simulink model "BCI_Control_Log_2024a"  (R2024a)
settings: Solver=FixedStepAuto  StartTime=0.0  StopTime=inf  FixedStep=1/fs  RelTol=1e-3
InitFcn:
  | RunTime
StopFcn:
  | SaveData
values from neighbouring files (symbols this model uses):
  const_a = Mdl_a.Coeffs(1,2).Const    [RunTime.m]
  ERaw = data{1,1}.X'    [RunTime.m]
  fs = 250    [SaveData.m]    (also in setup.m)
  ind_sel_a = Ia    [OfflineDataAnalysis_Unicorn.m]    (also in RunTime.m = Ia(1:best_feat_a))
  linear_coeffs_a = Mdl_a.Coeffs(1,2).Linear    [RunTime.m]
  shiftLen = 0.20*fs    [RunTime.m]
  winLen = 2*fs    [RunTime.m]
undefined symbols (not defined in the file or in its folder): UN, W1a, W2a
libraries: dspfdesign x34, dspnetwork x4, dspstat3 x2, UnicornLib x1
settings Model: Creator=Utente  LastModifiedBy=IRISc
settings DebuggingCC: UnconnectedInputMsg=warning  UnconnectedOutputMsg=warning  UnconnectedLineMsg=warning
settings ModelReferenceCC: EnableRefExpFcnMdlSchedulingChecks=on
settings RTWCC: GPUComputeCapability=3.5  DLArmComputeVersion=19.05

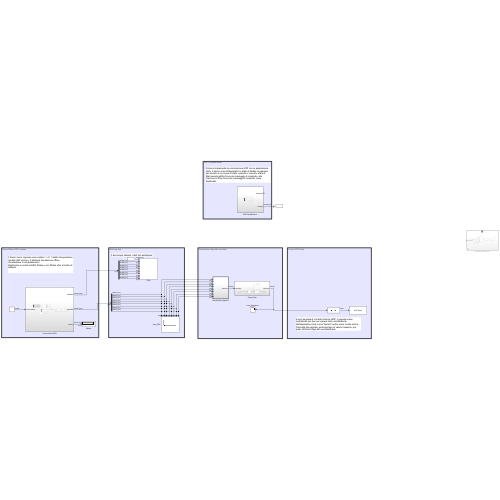
[thumbnail: Simulink's stored preview of the top-level diagram]
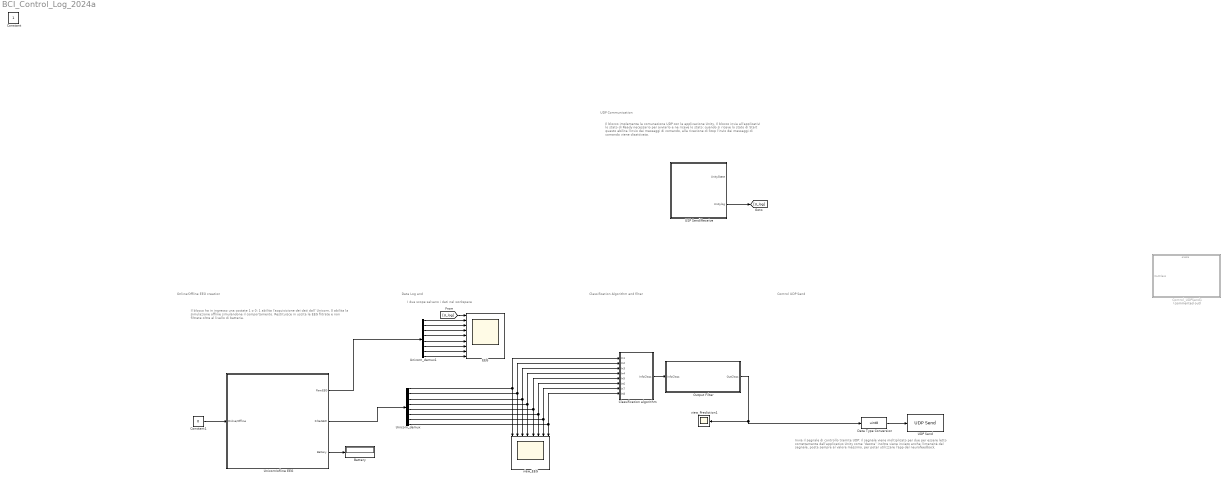
== system BCI_Control_Log_2024a ==
  note: Invia il segnale di controllo tramite UDP: il segnale viene moltiplicato per due per essere letto correttamente dall'applicativo Unity come "destra" inoltre viene inviato anche l'intensità del segnale, posta sempre al valore massimo, per poter utilizzare l'app del neurofeedback.
  note: Control UDP Send
  note: Il blocco implementa la comunazione UDP con le applicazione Unity. Il blocco invia all'applicativi lo stato di Ready necessario per avviarlo e ne riceve lo stato: quando si riceve lo stato di Start questo abilita l'invio dei messaggi di comando, alla ricezione di Stop l'invio dei messaggi di comando viene disattivata.
  note: UDP Communication
  note: Classification Algorithm and filter
  note: I due scope salvano i dati nel workspace
  note: Data Log and
  note: Il blocco ha in ingresso una costate 1 o 0: 1 abilita l'acquisizione dei dati dall' Unicorn, 0 abilita la simulazione offline simulandone il comportamento.
      | Restituisce in uscita le EEG flitrate e non filtrate oltre al livello di batteria.
  note: Online/Offline EEG creation
  Battery : Display
  Classification algorithm : Subsystem  TreatAsAtomicUnit=on
  Constant1 : Constant  Value=0
  Control_UDPSend1 : Subsystem  Commented=on
  Data Type Conversion : DataTypeConversion  OutDataTypeStr=uint8  SaturateOnIntegerOverflow=off  RndMeth=Floor
  EEG : Scope  NumInputPorts=9
  Output Filter : Subsystem
  UDP Send : dspnetwork/UDP Send  remoteURL='127.0.0.1'  remotePort=5010  localURL='0.0.0.0'  localPortSource=Automatically determine  localPort=-1  sendBufferSize=8192  sampletime=-1  blockPlatform=[]  separateLengthPort=0
  "USP Send/Receive " : Subsystem
  Unicorn/ofline EEG : Subsystem
  Unicorn_demux : Demux  Outputs=8
  Unicorn_demux1 : Demux  Outputs=8
  view_EEG : Scope  NumInputPorts=8
  view_Prediction1 : Scope
  Constant : Constant  IOType=siggen
  wires:
  Unicorn_demux/8 -> Classification algorithm/8(In8), view_EEG/8
  Unicorn_demux/7 -> Classification algorithm/7(In7), view_EEG/7
  Unicorn_demux/6 -> Classification algorithm/6(In6), view_EEG/6
  Unicorn_demux/5 -> Classification algorithm/5(In5), view_EEG/5
  Unicorn_demux/4 -> Classification algorithm/4(In4), view_EEG/4
  Unicorn_demux/1 -> Classification algorithm/1(In1), view_EEG/1
  Unicorn_demux/2 -> Classification algorithm/2(In2), view_EEG/2
  Unicorn_demux/3 -> Classification algorithm/3(In3), view_EEG/3
  Classification algorithm/1(InfoClass) -> Output Filter/1(InfoClass)
  Output Filter/1(OutClass) -> Data Type Conversion/1, view_Prediction1/1
  Unicorn/ofline EEG/2(FilterEEG) -> Unicorn_demux/1
  Unicorn/ofline EEG/1(RawEEG) -> Unicorn_demux1/1
  Unicorn/ofline EEG/3(Battery) -> Battery/1
  Constant1/1 -> Unicorn/ofline EEG/1(Online/Offline)
  Unicorn_demux1/1 -> EEG/2
  Unicorn_demux1/2 -> EEG/3
  Unicorn_demux1/3 -> EEG/4
  Unicorn_demux1/4 -> EEG/5
  Unicorn_demux1/5 -> EEG/6
  Unicorn_demux1/6 -> EEG/7
  Unicorn_demux1/7 -> EEG/8
  Unicorn_demux1/8 -> EEG/9
  "USP Send/Receive "/2(Unitylog) -> [U_log]
  [U_log] -> EEG/1
  Data Type Conversion/1 -> UDP Send/1

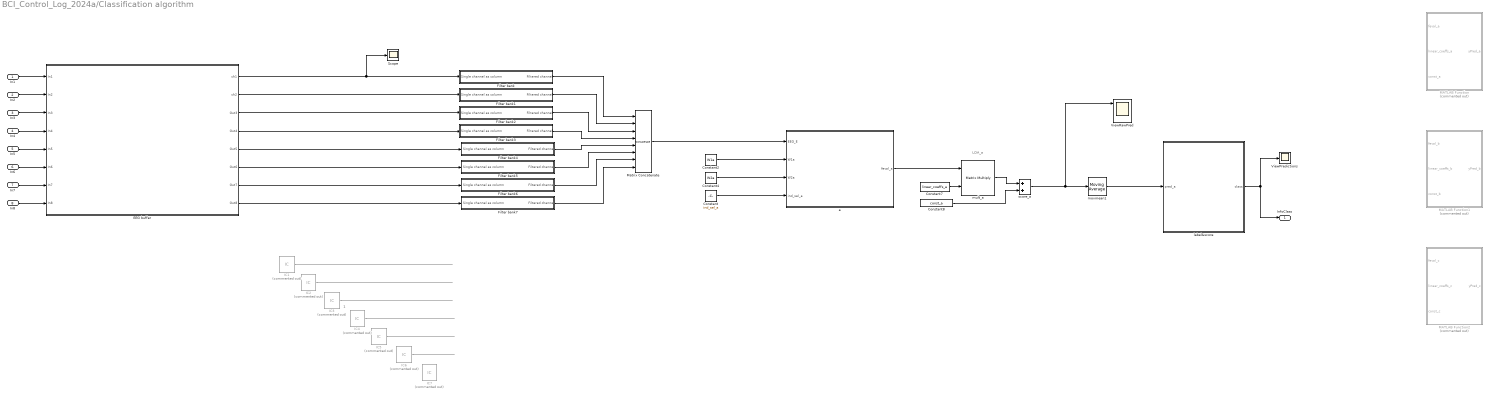
== system BCI_Control_Log_2024a/Classification algorithm ==
  note: LDA_a
  note: 1
  In1 : Inport
  In2 : Inport  Port=2
  In3 : Inport  Port=3
  In4 : Inport  Port=4
  In5 : Inport  Port=5
  In6 : Inport  Port=6
  In7 : Inport  Port=7
  In8 : Inport  Port=8
  Constant : Constant  Value=ind_sel_a
  Constant2 : Constant  Value=W1a
  Constant4 : Constant  Value=W2a
  Constant7 : Constant  Value=linear_coeffs_a
  Constant8 : Constant  Value=const_a
  EEG buffer : Subsystem
  Filter bank : Subsystem
  Filter bank1 : Subsystem
  Filter bank2 : Subsystem
  Filter bank3 : Subsystem
  Filter bank4 : Subsystem
  Filter bank5 : Subsystem
  Filter bank6 : Subsystem
  Filter bank7 : Subsystem
  IC{1..7} (7 alike) : InitialCondition  Commented=on  Value=0.1
  MATLAB Function : MATLAB Function  Commented=on  TreatAsAtomicUnit=on
  MATLAB Function1 : MATLAB Function  Commented=on  TreatAsAtomicUnit=on
  MATLAB Function2 : MATLAB Function  Commented=on  TreatAsAtomicUnit=on
  Matrix Concatenate : Concatenate  NumInputs=8  Mode=Multidimensional array  ConcatenateDimension=3
  Scope : Scope
  ViewPredictions : Scope
  ViewRawPred : Scope  NumInputPorts=3
  a : MATLAB Function  TreatAsAtomicUnit=on
  label&score : MATLAB Function  TreatAsAtomicUnit=on
  movmean1 : dspstat3/Moving Average  Method=Sliding window  ForgettingFactorPort=off  SpecifyWindowLength=on  WindowLength=3  OverlapLength=2  AllowArbitraryInputLength=off  ForgettingFactor=0.9  SimulateUsing=Code generation
  mult_a : Product  Multiplication=Matrix(*)
  score_a : Sum
  InfoClass : Outport
  wires:
  In1/1 -> EEG buffer/1(In1)
  In2/1 -> EEG buffer/2(In2)
  In3/1 -> EEG buffer/3(In3)
  In4/1 -> EEG buffer/4(In4)
  In5/1 -> EEG buffer/5(In5)
  In6/1 -> EEG buffer/6(In6)
  In7/1 -> EEG buffer/7(In7)
  In8/1 -> EEG buffer/8(In8)
  EEG buffer/1(ch1) -> Scope/1, Filter bank/1(Single channel as column)
  label&score/1(class) -> ViewPredictions/1, InfoClass/1
  Filter bank5/1(Filtered channel) -> Matrix Concatenate/6
  Filter bank6/1(Filtered channel) -> Matrix Concatenate/7
  a/1(feval_a) -> mult_a/1
  Filter bank4/1(Filtered channel) -> Matrix Concatenate/5
  Filter bank1/1(Filtered channel) -> Matrix Concatenate/2
  Filter bank7/1(Filtered channel) -> Matrix Concatenate/8
  Filter bank2/1(Filtered channel) -> Matrix Concatenate/3
  Filter bank3/1(Filtered channel) -> Matrix Concatenate/4
  Filter bank/1(Filtered channel) -> Matrix Concatenate/1
  Matrix Concatenate/1 -> a/1(EEG_E)
  EEG buffer/8(Out8) -> Filter bank7/1(Single channel as column)
  Constant/1 -> a/4(ind_sel_a)
  Constant4/1 -> a/3(W2a)
  Constant2/1 -> a/2(W1a)
  Constant7/1 -> mult_a/2
  Constant8/1 -> score_a/2
  score_a/1 -> ViewRawPred/1, movmean1/1
  mult_a/1 -> score_a/1
  IC1/1 -> ?
  IC4/1 -> ?
  ? -> IC6/1
  IC2/1 -> ?
  ? -> IC2/1
  IC5/1 -> ?
  ? -> IC5/1
  ? -> IC7/1
  ? -> IC4/1
  IC3/1 -> ?
  ? -> IC1/1
  IC6/1 -> ?
  ? -> IC3/1
  EEG buffer/2(ch2) -> Filter bank1/1(Single channel as column)
  EEG buffer/3(Out3) -> Filter bank2/1(Single channel as column)
  EEG buffer/4(Out4) -> Filter bank3/1(Single channel as column)
  EEG buffer/5(Out5) -> Filter bank4/1(Single channel as column)
  EEG buffer/6(Out6) -> Filter bank5/1(Single channel as column)
  EEG buffer/7(Out7) -> Filter bank6/1(Single channel as column)
  movmean1/1 -> label&score/1(pred_a)

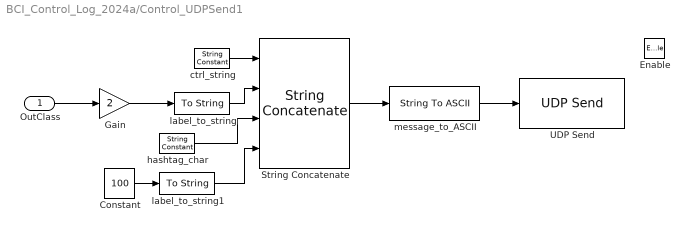
== system BCI_Control_Log_2024a/Control_UDPSend1 ==
  OutClass : Inport
  Enable : EnablePort
  Constant : Constant  Value=100
  Gain : Gain  Gain=2
  String Concatenate : StringConcatenate  Inputs=4
  UDP Send : dspnetwork/UDP Send  remoteURL='127.0.0.1'  remotePort=8000  localURL='0.0.0.0'  localPortSource=Automatically determine  localPort=-1  sendBufferSize=8192  sampletime=-1  blockPlatform=[]  separateLengthPort=0
  ctrl_string : StringConstant  String="\"ctrl#\""
  hashtag_char : StringConstant  String="\"#\""
  label_to_string : ToString
  label_to_string1 : ToString
  message_to_ASCII : StringToASCII
  wires:
  String Concatenate/1 -> message_to_ASCII/1
  label_to_string/1 -> String Concatenate/2
  OutClass/1 -> Gain/1
  ctrl_string/1 -> String Concatenate/1
  message_to_ASCII/1 -> UDP Send/1
  hashtag_char/1 -> String Concatenate/3
  Constant/1 -> label_to_string1/1
  label_to_string1/1 -> String Concatenate/4
  Gain/1 -> label_to_string/1

== system BCI_Control_Log_2024a/Output Filter ==
  InfoClass : Inport
  MATLAB Function1 : MATLAB Function  TreatAsAtomicUnit=on
  Moving Average : dspstat3/Moving Average  Method=Sliding window  ForgettingFactorPort=off  SpecifyWindowLength=on  WindowLength=7  OverlapLength=6  AllowArbitraryInputLength=off  ForgettingFactor=0.9  SimulateUsing=Interpreted execution
  Scope : Scope
  OutClass : Outport
  wires:
  Moving Average/1 -> Scope/1, MATLAB Function1/1(u)
  MATLAB Function1/1(y) -> OutClass/1
  InfoClass/1 -> Moving Average/1

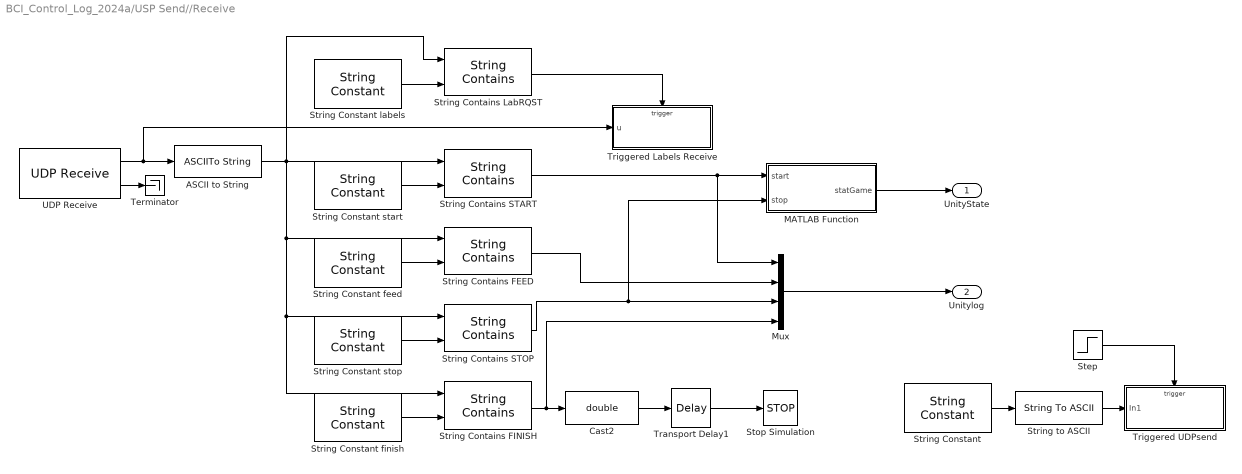
== system BCI_Control_Log_2024a/USP Send//Receive  ==
  ASCII to String : ASCIIToString
  Cast2 : DataTypeConversion  OutDataTypeStr=double  SaturateOnIntegerOverflow=off  RndMeth=Floor
  MATLAB Function : MATLAB Function  TreatAsAtomicUnit=on
  Mux : Mux
  Step : Step  SampleTime=1/fs
  Stop Simulation : Stop
  String Constant : StringConstant  String="\"ready#\""
  String Constant feed : StringConstant  String="\"feed\""
  String Constant finish : StringConstant  String="\"finish\""
  String Constant labels : StringConstant  String="\"labels#\""
  String Constant start : StringConstant  String="\"start\""
  String Constant stop : StringConstant  String="\"stop\""
  String Contains FEED : StringContains
  String Contains FINISH : StringContains
  String Contains LabRQST : StringContains
  String Contains START : StringContains
  String Contains STOP : StringContains
  String to ASCII : StringToASCII
  Terminator : Terminator
  Transport Delay1 : TransportDelay
  Triggered Labels Receive : Subsystem  TreatAsAtomicUnit=on
  Triggered UDPsend : Subsystem  TreatAsAtomicUnit=on
  UDP Receive : dspnetwork/UDP Receive  localURL='0.0.0.0'  localPort=8001  remoteURL='0.0.0.0'  remotePort=-1  recvBufferSize=8192  dims=255  signalDatatype=uint8  isComplex=off  isVarSize=off  showBlockingTime=off  blockingTime=0  sampletime=-1  blockPlatform=[]
  UnityState : Outport
  Unitylog : Outport  Port=2
  wires:
  Cast2/1 -> Transport Delay1/1
  Transport Delay1/1 -> Stop Simulation/1
  String Constant/1 -> String to ASCII/1
  String Contains LabRQST/1 -> Triggered Labels Receive/Trigger
  UDP Receive/2 -> Terminator/1
  String Constant feed/1 -> String Contains FEED/2
  String Constant stop/1 -> String Contains STOP/2
  String Constant start/1 -> String Contains START/2
  String Contains FINISH/1 -> Mux/4, Cast2/1
  String Contains FEED/1 -> Mux/2
  String Contains START/1 -> Mux/1, MATLAB Function/1(start)
  ASCII to String/1 -> String Contains FINISH/1, String Contains STOP/1, String Contains FEED/1, String Contains LabRQST/1, String Contains START/1
  String to ASCII/1 -> Triggered UDPsend/1(In1)
  Step/1 -> Triggered UDPsend/Trigger
  UDP Receive/1 -> Triggered Labels Receive/1(u), ASCII to String/1
  String Constant labels/1 -> String Contains LabRQST/2
  String Constant finish/1 -> String Contains FINISH/2
  MATLAB Function/1(statGame) -> UnityState/1
  String Contains STOP/1 -> Mux/3, MATLAB Function/2(stop)
  Mux/1 -> Unitylog/1

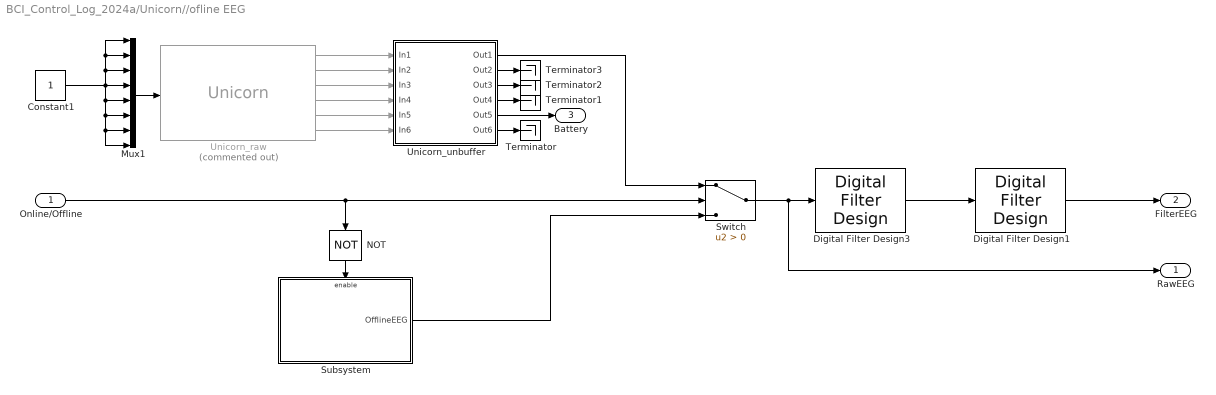
== system BCI_Control_Log_2024a/Unicorn//ofline EEG ==
  Online/Offline : Inport
  Constant1 : Constant  OutDataTypeStr=boolean
  Digital Filter Design1 : dspfdesign/Digital Filter Design  mwdsp_browser_bugfix_var=off
  Digital Filter Design3 : dspfdesign/Digital Filter Design  mwdsp_browser_bugfix_var=off
  Mux1 : Mux  Inputs=8
  NOT : Logic  Operator=NOT  IconShape=distinctive  AllPortsSameDT=off  OutDataTypeStr=boolean
  Subsystem : Subsystem
  Switch : Switch  Criteria=u2 > Threshold  SaturateOnIntegerOverflow=off  InputSameDT=off
  Terminator{,1..3} (4 alike) : Terminator
  Unicorn_raw : UnicornLib/Unicorn  Commented=on  serial=UN-2023.04.40  old_serial=UN-2023.04.40  frame_length=1  input_source=Electrode
      settings: SourceProductName=Unicorn
  Unicorn_unbuffer : Subsystem
      mask Display:
      | port_label('input',1,'EEG')
      | port_label('input',2,'ACC')
      | port_label('input',3,'GYRO')
      | port_label('input',4,'VALID')
      | port_label('input',5,'BAT')
      | port_label('input',6,'CNT')
      | port_label('output',1,'EEG')
      | port_label('output',2,'ACC')
      | port_label('output',3,'GYRO')
      | port_label('output',4,'VALID')
      | port_label('output',5,'BAT')
      | port_label('output',6,'CNT')
  RawEEG : Outport
  FilterEEG : Outport  Port=2
  Battery : Outport  Port=3
  wires:
  Subsystem/1(OfflineEEG) -> Switch/3
  Mux1/1 -> Unicorn_raw/1
  Unicorn_raw/1 -> Unicorn_unbuffer/1(In1)
  Unicorn_raw/3 -> Unicorn_unbuffer/3(In3)
  Unicorn_raw/5 -> Unicorn_unbuffer/5(In5)
  Digital Filter Design1/1 -> FilterEEG/1
  Unicorn_unbuffer/2(Out2) -> Terminator3/1
  Constant1/1 -> Mux1/2, Mux1/1, Mux1/3, Mux1/5, Mux1/6, Mux1/7, Mux1/8, Mux1/4
  Unicorn_raw/2 -> Unicorn_unbuffer/2(In2)
  Unicorn_raw/4 -> Unicorn_unbuffer/4(In4)
  Unicorn_unbuffer/4(Out4) -> Terminator1/1
  Unicorn_unbuffer/6(Out6) -> Terminator/1
  Digital Filter Design3/1 -> Digital Filter Design1/1
  Unicorn_unbuffer/3(Out3) -> Terminator2/1
  Unicorn_raw/6 -> Unicorn_unbuffer/6(In6)
  Online/Offline/1 -> NOT/1, Switch/2
  Unicorn_unbuffer/1(Out1) -> Switch/1
  Switch/1 -> RawEEG/1, Digital Filter Design3/1
  Unicorn_unbuffer/5(Out5) -> Battery/1
  NOT/1 -> Subsystem/Enable

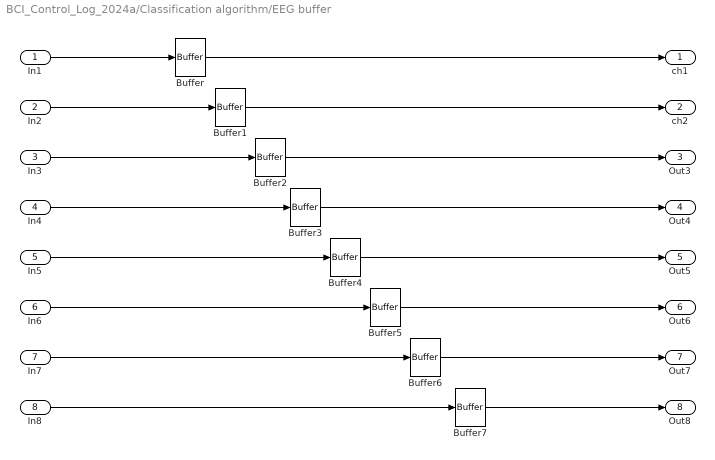
== system BCI_Control_Log_2024a/Classification algorithm/EEG buffer ==
  In1 : Inport
  In2 : Inport  Port=2
  In3 : Inport  Port=3
  In4 : Inport  Port=4
  In5 : Inport  Port=5
  In6 : Inport  Port=6
  In7 : Inport  Port=7
  In8 : Inport  Port=8
  Buffer{,1..7} (8 alike) : Buffer  N=winLen  V=winLen-floor(shiftLen)  OutputFrames=off
  ch1 : Outport
  ch2 : Outport  Port=2
  Out3 : Outport  Port=3
  Out4 : Outport  Port=4
  Out5 : Outport  Port=5
  Out6 : Outport  Port=6
  Out7 : Outport  Port=7
  Out8 : Outport  Port=8
  wires:
  Buffer/1 -> ch1/1
  In4/1 -> Buffer3/1
  In3/1 -> Buffer2/1
  In5/1 -> Buffer4/1
  Buffer5/1 -> Out6/1
  In1/1 -> Buffer/1
  In2/1 -> Buffer1/1
  Buffer7/1 -> Out8/1
  In7/1 -> Buffer6/1
  Buffer2/1 -> Out3/1
  In8/1 -> Buffer7/1
  Buffer4/1 -> Out5/1
  In6/1 -> Buffer5/1
  Buffer1/1 -> ch2/1
  Buffer3/1 -> Out4/1
  Buffer6/1 -> Out7/1

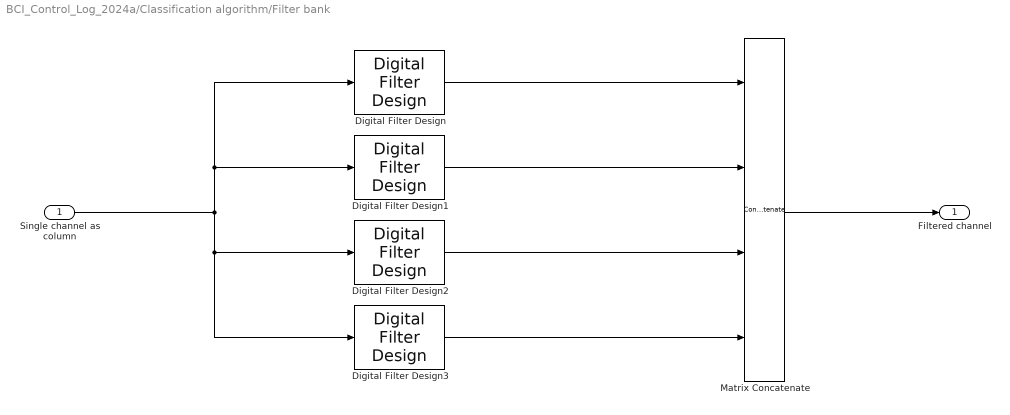
== system BCI_Control_Log_2024a/Classification algorithm/Filter bank ==
  Single channel as column : Inport
  Digital Filter Design{,1..3} (4 alike) : dspfdesign/Digital Filter Design  mwdsp_browser_bugfix_var=off
  Matrix Concatenate : Concatenate  NumInputs=4  Mode=Multidimensional array  ConcatenateDimension=2
  Filtered channel : Outport  VectorParamsAs1DForOutWhenUnconnected=off
  wires:
  Digital Filter Design1/1 -> Matrix Concatenate/2
  Digital Filter Design3/1 -> Matrix Concatenate/4
  Single channel as column/1 -> Digital Filter Design1/1, Digital Filter Design/1, Digital Filter Design3/1, Digital Filter Design2/1
  Digital Filter Design/1 -> Matrix Concatenate/1
  Digital Filter Design2/1 -> Matrix Concatenate/3
  Matrix Concatenate/1 -> Filtered channel/1

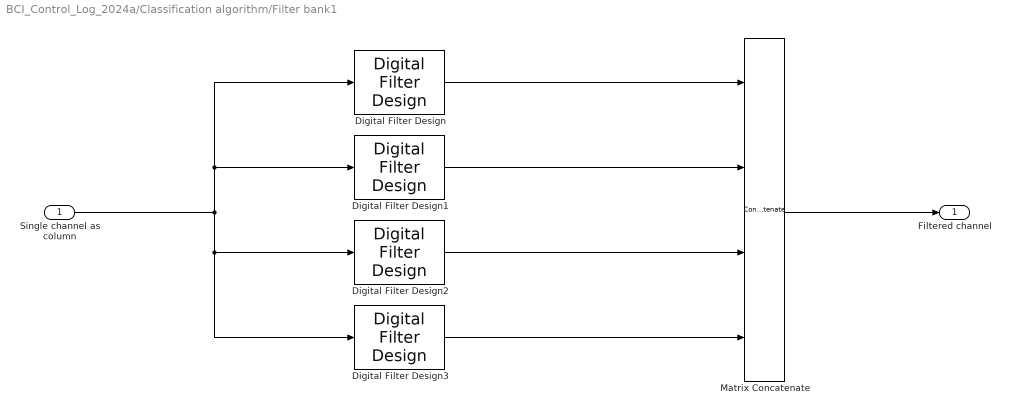
== system BCI_Control_Log_2024a/Classification algorithm/Filter bank1 ==
  Single channel as column : Inport
  Digital Filter Design{,1..3} (4 alike) : dspfdesign/Digital Filter Design  mwdsp_browser_bugfix_var=off
  Matrix Concatenate : Concatenate  NumInputs=4  Mode=Multidimensional array  ConcatenateDimension=2
  Filtered channel : Outport  VectorParamsAs1DForOutWhenUnconnected=off
  wires:
  Digital Filter Design1/1 -> Matrix Concatenate/2
  Digital Filter Design3/1 -> Matrix Concatenate/4
  Single channel as column/1 -> Digital Filter Design/1, Digital Filter Design1/1, Digital Filter Design2/1, Digital Filter Design3/1
  Digital Filter Design/1 -> Matrix Concatenate/1
  Digital Filter Design2/1 -> Matrix Concatenate/3
  Matrix Concatenate/1 -> Filtered channel/1

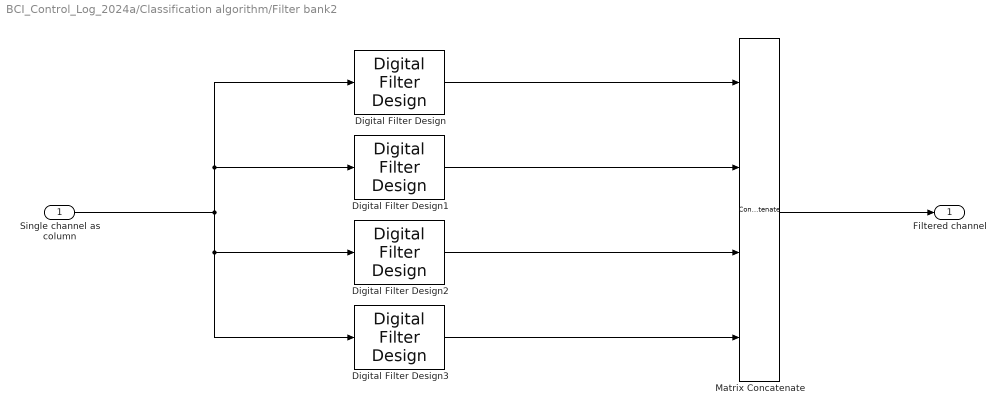
== system BCI_Control_Log_2024a/Classification algorithm/Filter bank2 ==
  Single channel as column : Inport
  Digital Filter Design{,1..3} (4 alike) : dspfdesign/Digital Filter Design  mwdsp_browser_bugfix_var=off
  Matrix Concatenate : Concatenate  NumInputs=4  Mode=Multidimensional array  ConcatenateDimension=2
  Filtered channel : Outport  VectorParamsAs1DForOutWhenUnconnected=off
  wires:
  Matrix Concatenate/1 -> Filtered channel/1
  Single channel as column/1 -> Digital Filter Design1/1, Digital Filter Design/1, Digital Filter Design3/1, Digital Filter Design2/1
  Digital Filter Design/1 -> Matrix Concatenate/1
  Digital Filter Design3/1 -> Matrix Concatenate/4
  Digital Filter Design2/1 -> Matrix Concatenate/3
  Digital Filter Design1/1 -> Matrix Concatenate/2

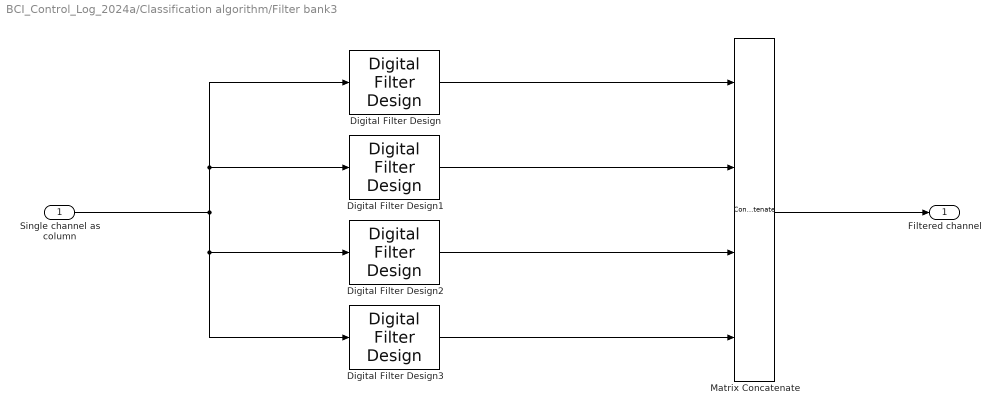
== system BCI_Control_Log_2024a/Classification algorithm/Filter bank3 ==
  Single channel as column : Inport
  Digital Filter Design{,1..3} (4 alike) : dspfdesign/Digital Filter Design  mwdsp_browser_bugfix_var=off
  Matrix Concatenate : Concatenate  NumInputs=4  Mode=Multidimensional array  ConcatenateDimension=2
  Filtered channel : Outport  VectorParamsAs1DForOutWhenUnconnected=off
  wires:
  Matrix Concatenate/1 -> Filtered channel/1
  Single channel as column/1 -> Digital Filter Design1/1, Digital Filter Design/1, Digital Filter Design2/1, Digital Filter Design3/1
  Digital Filter Design/1 -> Matrix Concatenate/1
  Digital Filter Design3/1 -> Matrix Concatenate/4
  Digital Filter Design2/1 -> Matrix Concatenate/3
  Digital Filter Design1/1 -> Matrix Concatenate/2

== system BCI_Control_Log_2024a/Classification algorithm/Filter bank4 ==
  Single channel as column : Inport
  Digital Filter Design{,1..3} (4 alike) : dspfdesign/Digital Filter Design  mwdsp_browser_bugfix_var=off
  Matrix Concatenate : Concatenate  NumInputs=4  Mode=Multidimensional array  ConcatenateDimension=2
  Filtered channel : Outport  VectorParamsAs1DForOutWhenUnconnected=off
  wires:
  Matrix Concatenate/1 -> Filtered channel/1
  Single channel as column/1 -> Digital Filter Design/1, Digital Filter Design1/1, Digital Filter Design2/1, Digital Filter Design3/1
  Digital Filter Design/1 -> Matrix Concatenate/1
  Digital Filter Design3/1 -> Matrix Concatenate/4
  Digital Filter Design2/1 -> Matrix Concatenate/3
  Digital Filter Design1/1 -> Matrix Concatenate/2

== system BCI_Control_Log_2024a/Classification algorithm/Filter bank5 ==
  Single channel as column : Inport
  Digital Filter Design{,1..3} (4 alike) : dspfdesign/Digital Filter Design  mwdsp_browser_bugfix_var=off
  Matrix Concatenate : Concatenate  NumInputs=4  Mode=Multidimensional array  ConcatenateDimension=2
  Filtered channel : Outport  VectorParamsAs1DForOutWhenUnconnected=off
  wires:
  Matrix Concatenate/1 -> Filtered channel/1
  Single channel as column/1 -> Digital Filter Design1/1, Digital Filter Design/1, Digital Filter Design2/1, Digital Filter Design3/1
  Digital Filter Design/1 -> Matrix Concatenate/1
  Digital Filter Design3/1 -> Matrix Concatenate/4
  Digital Filter Design2/1 -> Matrix Concatenate/3
  Digital Filter Design1/1 -> Matrix Concatenate/2

== system BCI_Control_Log_2024a/Classification algorithm/Filter bank6 ==
  Single channel as column : Inport
  Digital Filter Design{,1..3} (4 alike) : dspfdesign/Digital Filter Design  mwdsp_browser_bugfix_var=off
  Matrix Concatenate1 : Concatenate  NumInputs=4  Mode=Multidimensional array  ConcatenateDimension=2
  Filtered channel : Outport  VectorParamsAs1DForOutWhenUnconnected=off
  wires:
  Matrix Concatenate1/1 -> Filtered channel/1
  Single channel as column/1 -> Digital Filter Design1/1, Digital Filter Design/1, Digital Filter Design3/1, Digital Filter Design2/1
  Digital Filter Design/1 -> Matrix Concatenate1/1
  Digital Filter Design3/1 -> Matrix Concatenate1/4
  Digital Filter Design2/1 -> Matrix Concatenate1/3
  Digital Filter Design1/1 -> Matrix Concatenate1/2

== system BCI_Control_Log_2024a/Classification algorithm/Filter bank7 ==
  Single channel as column : Inport
  Digital Filter Design{,1..3} (4 alike) : dspfdesign/Digital Filter Design  mwdsp_browser_bugfix_var=off
  Matrix Concatenate : Concatenate  NumInputs=4  Mode=Multidimensional array  ConcatenateDimension=2
  Filtered channel : Outport  VectorParamsAs1DForOutWhenUnconnected=off
  wires:
  Matrix Concatenate/1 -> Filtered channel/1
  Single channel as column/1 -> Digital Filter Design1/1, Digital Filter Design/1, Digital Filter Design3/1, Digital Filter Design2/1
  Digital Filter Design/1 -> Matrix Concatenate/1
  Digital Filter Design3/1 -> Matrix Concatenate/4
  Digital Filter Design2/1 -> Matrix Concatenate/3
  Digital Filter Design1/1 -> Matrix Concatenate/2

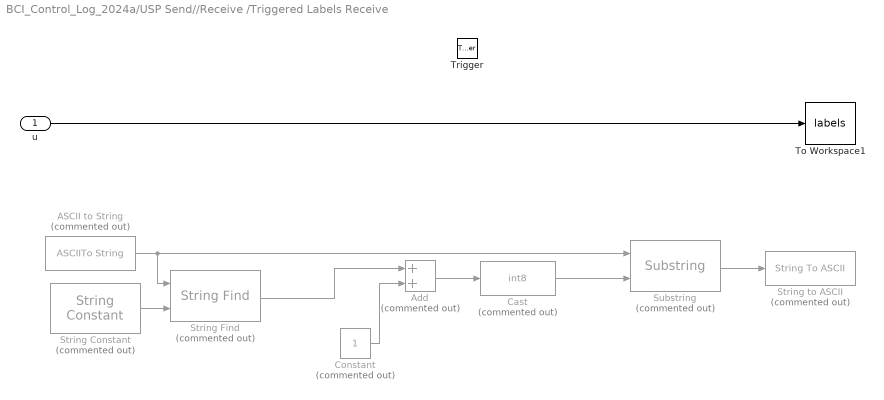
== system BCI_Control_Log_2024a/USP Send//Receive /Triggered Labels Receive ==
  u : Inport
  Trigger : TriggerPort  VariantControl=Variant  PortDimensions=1
  ASCII to String : ASCIIToString  Commented=on
  Add : Sum  Commented=on
  Cast : DataTypeConversion  Commented=on  OutDataTypeStr=int8  SaturateOnIntegerOverflow=off  RndMeth=Floor
  Constant : Constant  Commented=on
  String Constant : StringConstant  Commented=on  String="\"#\""
  String Find : StringFind  Commented=on
  String to ASCII : StringToASCII  Commented=on
  Substring : Substring  Commented=on  StringFromIdxToEnd=on
  To Workspace1 : ToWorkspace  VariableName=labels  SampleTime=-1
      settings: Save2DSignal=2-D array (concatenate along first dimension)
  wires:
  u/1 -> To Workspace1/1
  Add/1 -> Cast/1
  Cast/1 -> Substring/2
  ASCII to String/1 -> String Find/1, Substring/1
  String Constant/1 -> String Find/2
  String Find/1 -> Add/1
  Substring/1 -> String to ASCII/1
  Constant/1 -> Add/2

== system BCI_Control_Log_2024a/USP Send//Receive /Triggered UDPsend ==
  In1 : Inport
  Trigger : TriggerPort  VariantControl=Variant
  UDP Send : dspnetwork/UDP Send  remoteURL='127.0.0.1'  remotePort=8000  localURL='0.0.0.0'  localPortSource=Automatically determine  localPort=-1  sendBufferSize=8192  sampletime=-1  blockPlatform=[]  separateLengthPort=0
  wires:
  In1/1 -> UDP Send/1

== system BCI_Control_Log_2024a/Unicorn//ofline EEG/Subsystem ==
  Online/Offline : EnablePort
  test_RawEEG1 : Constant  Value=ERaw  SampleTime=(1/fs)*length(ERaw)
  tranpose_test1 : Math  Operator=transpose
  unbuffer_test1 : Unbuffer
  OfflineEEG : Outport
  wires:
  test_RawEEG1/1 -> tranpose_test1/1
  tranpose_test1/1 -> unbuffer_test1/1
  unbuffer_test1/1 -> OfflineEEG/1

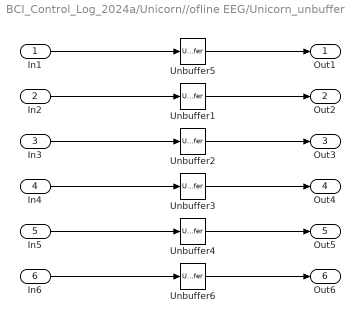
== system BCI_Control_Log_2024a/Unicorn//ofline EEG/Unicorn_unbuffer ==
  In1 : Inport
  In2 : Inport  Port=2
  In3 : Inport  Port=3
  In4 : Inport  Port=4
  In5 : Inport  Port=5
  In6 : Inport  Port=6
  Unbuffer{1..6} (6 alike) : Unbuffer
  Out1 : Outport
  Out2 : Outport  Port=2
  Out3 : Outport  Port=3
  Out4 : Outport  Port=4
  Out5 : Outport  Port=5
  Out6 : Outport  Port=6
  wires:
  In2/1 -> Unbuffer1/1
  In3/1 -> Unbuffer2/1
  In4/1 -> Unbuffer3/1
  In5/1 -> Unbuffer4/1
  Unbuffer4/1 -> Out5/1
  Unbuffer3/1 -> Out4/1
  Unbuffer2/1 -> Out3/1
  Unbuffer1/1 -> Out2/1
  Unbuffer6/1 -> Out6/1
  In6/1 -> Unbuffer6/1
  In1/1 -> Unbuffer5/1
  Unbuffer5/1 -> Out1/1

== matlab function BCI_Control_Log_2024a/Classification algorithm/label&score ==
  data: pred_a input; class output
function class = get_class(pred_a)
    % Se il punteggio è positivo o zero, Movimento
    if pred_a >= 0 
        class = 1; 
    % Se il punteggio è negativo, Riposo
    else
        class = 0; 
    end
end

%codice di prima faceva se pred_a>0 e pred_b>0 allora sicuro era sinistra
% classificatore A dice che sei a destra della sua linea E il classificatore B
% dice che sei a destra della sua linea... allora incrociando i dati sei sicuramente la classe Sinistra

% function class = get_class(pred_a, pred_b, pred_c)
%     if ((pred_a>=0) && (pred_b>=0)) %1 left
%         class = -1;
%     elseif ((pred_a<0) && (pred_c>=0)) %2 right
%         class= 1;
%     else %rest
%         class = 0;
%     end
% end


% function class = get_class(pred_a, pred_b, pred_c)
% 
% if ((pred_a==1) && (pred_b==1)) %1 left
%     class = -1;
% elseif ((pred_a==2) && (pred_c==2)) %2 right
%     class= 1;
% else %rest
%     class = 0;
% end
% 
% 
% end

== matlab function BCI_Control_Log_2024a/Classification algorithm/a ==
  data: EEG_E input; feval_a output; W1a input; W2a input; ind_sel_a input
function feval_a = CSPeval_a(EEG_E,W1a,W2a,ind_sel_a)

EEG_E = permute(EEG_E,[3,1,2]); %dim [8 x 500 x 4]

% CSP

V1a_eval  = CSPapply(EEG_E,[],W1a,W2a,[],[]);

feval_a = V1a_eval(:,ind_sel_a);
% else
%     V1a_eval = zeros(1,24)
% 
%     feval_a = V1a_eval(:,ind_sel_a)
% end


end

== matlab function BCI_Control_Log_2024a/Classification algorithm/MATLAB Function ==
  data: feval_a input; linear_coeffs_a input; yPred_a output; const_a input
% Calcola i punteggi discriminanti per ogni classe.
function yPred_a = ldaPredict_a(feval_a, linear_coeffs_a, const_a)
    % 'feval_a' è un vettore delle feature in ingresso
    % 'linear_coeffs_a' è una matrice dei coefficienti lineari
    % 'const_a' è un vettore dei bias (intercette)

    score = dot(feval_a, linear_coeffs_a) + const_a; 
    %score = linear_coeffs_a * feval_a + const_a;

    % Predizione: scegli la classe con il punteggio più alto
    if score > 0 
        yPred_a = 1;
    else
        yPred_a = 2;
    end
    
    %prova a dare in uscita lo score e poi lo confronti in get class come
    %fa MicSom
end

== matlab function BCI_Control_Log_2024a/Output Filter/MATLAB Function1 ==
  data: u input; y output
function y = fcn(u)
persistent u_back ;
u_back = 0 ;
if u >= u_back && u > 0.6
    u_back = u ;
    y = 1 ;
elseif u <= u_back && u < 0.6
    u_back = u ;
    y = 0 ;
elseif u > u_back
    u_back = u ;
    y = 0 ;
else
    u_back = u ;
    y = 1 ;
end

== matlab function BCI_Control_Log_2024a/Classification algorithm/MATLAB Function1 ==
  data: feval_b input; linear_coeffs_b input; yPred_b output; const_b input
% Calcola i punteggi discriminanti per ogni classe.
function yPred_b = ldaPredict_b(feval_b, linear_coeffs_b, const_b)
    % 'feval_a' è un vettore delle feature in ingresso
    % 'linear_coeffs_a' è una matrice dei coefficienti lineari
    % 'const_a' è un vettore dei bias (intercette)

    score = dot(feval_b, linear_coeffs_b) + const_b; 
    %score = linear_coeffs_b * feval_b + const_b;

    % Predizione: scegli la classe con il punteggio più alto
    if score > 0 
        yPred_b = 1;
    else
        yPred_b = 3;
    end
    
end

== matlab function BCI_Control_Log_2024a/Classification algorithm/MATLAB Function2 ==
  data: feval_c input; linear_coeffs_c input; yPred_c output; const_c input
% Calcola i punteggi discriminanti per ogni classe.
function yPred_c  = ldaPredict_c(feval_c, linear_coeffs_c, const_c)
    % 'feval_a' è un vettore delle feature in ingresso
    % 'linear_coeffs_a' è una matrice dei coefficienti lineari
    % 'const_a' è un vettore dei bias (intercette)

    score = dot(feval_c, linear_coeffs_c) + const_c; 
    %score = linear_coeffs_c * feval_c + const_c;

    % Predizione: scegli la classe con il punteggio più alto
    if score > 0 
        yPred_c = 2;
    else
        yPred_c = 3;
    end
    
end

== matlab function BCI_Control_Log_2024a/USP Send//Receive /MATLAB Function ==
  data: start input; statGame output; stop input
function statGame = start_stop(start, stop)

if start == 1
    statGame = 1;
elseif stop == 1
    %statGame= 2;
    statGame= 0;
else
    statGame = 0;

end
